simulink model "MSX60_10_by2"  (Simulink 7.9)
settings: Solver=ode14x  StartTime=0.0  StopTime=220  FixedStep=0.05  RelTol=1e-4
values from neighbouring files (symbols this model uses):
  G = yout(:,3)    [MSX60_10_by2_with_PandO.m]    (also in MSX60_10_by2_with_PandO_PS.m; MSX60_10_by2_with_PandO_US (1).m; MSX60_10_by2_with_PandO_US.m; MSX60_10by2Cell.m = 500)
  n = 1.3    [MSX60DS.m]    (also in MSX60_10_RL.m; MSX60_10_by2_with_PandO.m; MSX60_10_by2_with_PandO_PS.m; MSX60_10_by2_with_PandO_US (1).m)
  Ns = 1    [MSX60DS.m]    (also in MSX60_10_RL.m; MSX60_10_by2_with_PandO.m; MSX60_10_by2_with_PandO_PS.m; MSX60_10_by2_with_PandO_US (1).m)
  Rs = 0.58    [MSX60DS.m]    (also in MSX60_10_RL.m; MSX60_10_by2_with_PandO.m; MSX60_10_by2_with_PandO_PS.m; MSX60_10_by2_with_PandO_US (1).m)
  Voc = Voc(1)    [MSX60DS.m]    (also in MSX60_10_RL.m = 21.1; MSX60_10_by2_with_PandO.m = 21.1; MSX60_10_by2_with_PandO_PS.m = 21.1; MSX60_10_by2_with_PandO_US (1).m = 21.1)
libraries: fl_lib x23, elec_lib x20, nesl_utility x5, simulink x1
settings Model: Creator=pc1  LastModifiedBy=pc1
settings SolverCC: SolverJacobianMethodControl=SparsePerturbation
settings DataIOCC: SaveState=on

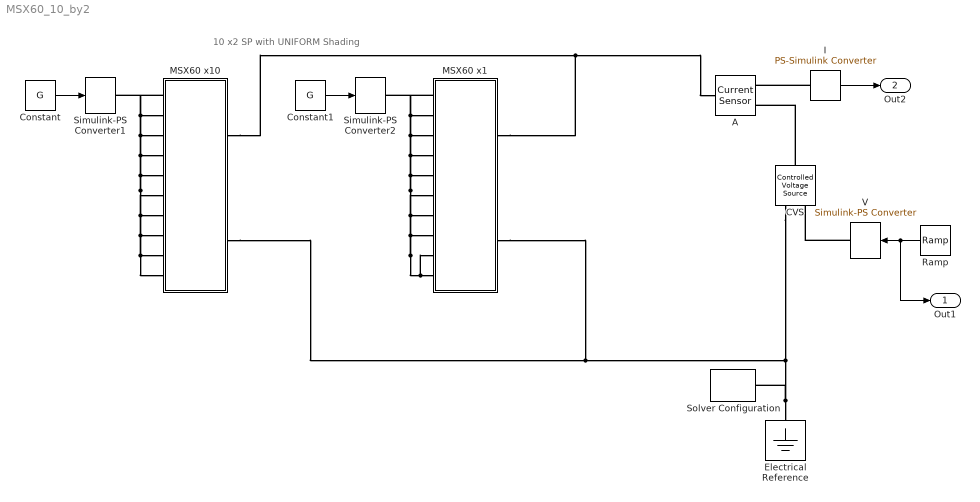
== system MSX60_10_by2 ==
  note: 10 x2 SP with UNIFORM Shading
  A : fl_lib/Electrical/Electrical Sensors/Current Sensor  i1_Log=off  v1_Log=off  LocalVarNames=|i1|v1  LocalVarDescs=|i1|v1  LocalVarLogging=[0 0]
  CVS : fl_lib/Electrical/Electrical Sources/Controlled Voltage Source  i_Log=off  v_Log=off  LocalVarNames=|i|v  LocalVarDescs=|i|v  LocalVarLogging=[0 0]
  Constant : Constant  Value=G
  Constant1 : Constant  Value=G
  Electrical Reference : fl_lib/Electrical/Electrical Elements/Electrical Reference  i_Log=off  LocalVarNames=|i  LocalVarDescs=|i  LocalVarLogging=0
  I : nesl_utility/PS-Simulink Converter  PhysicalDomain=network_engine_domain  LeftPortType=input  RightPortType=output  SubClassName=ps_output  Unit=1  AffineConversion=off
  MSX60 x1 : Subsystem
  MSX60 x10 : Subsystem
  Ramp : simulink/Sources/Ramp  slope=1  start=1  X0=0
  Simulink-PS Converter1 : nesl_utility/Simulink-PS Converter  PhysicalDomain=network_engine_domain  LeftPortType=input  RightPortType=output  SubClassName=ps_input  Unit=1  AffineConversion=off  InputFilterTimeConstant=.001  UdotUserProvided=[]  SimscapeFilterOrder=1  InputFiltering=off
  Simulink-PS Converter2 : nesl_utility/Simulink-PS Converter  PhysicalDomain=network_engine_domain  LeftPortType=input  RightPortType=output  SubClassName=ps_input  Unit=1  AffineConversion=off  InputFilterTimeConstant=.001  UdotUserProvided=[]  SimscapeFilterOrder=1  InputFiltering=off
  Solver Configuration : nesl_utility/Solver Configuration  PhysicalDomain=network_engine_domain  LeftPortType=input  RightPortType=generic  SubClassName=solver  UseCustomDae=off  DoDC=on  ResidualTolerance=1e-9  UseLocalSolver=off  LocalSolverChoice=NE_BACKWARD_EULER_ADVANCER  LocalSolverSampleTime=.001  DoFixedCost=off  MaxNonlinIter=3  MaxModeIter=2  LinearAlgebra=Sparse  Accelerate=off  Profile=off  UseLocalSampling=off  DelaysMemoryBudget=1024
  V : nesl_utility/Simulink-PS Converter  PhysicalDomain=network_engine_domain  LeftPortType=input  RightPortType=output  SubClassName=ps_input  Unit=1  AffineConversion=off  InputFilterTimeConstant=.001  UdotUserProvided=[]  SimscapeFilterOrder=1  InputFiltering=off
  Out1 : Outport
  Out2 : Outport  Port=2
  wires:
  I/1 -> Out2/1
  Ramp/1 -> V/1, Out1/1
  Constant/1 -> Simulink-PS Converter1/1
  Constant1/1 -> Simulink-PS Converter2/1
  connections:
  I/LConn1 -- A/RConn1
  MSX60 x10/RConn2 -- CVS/RConn2 -- Electrical Reference/LConn1 -- Solver Configuration/RConn1 -- MSX60 x1/RConn2
  CVS/LConn1 -- A/RConn2
  V/RConn1 -- CVS/RConn1
  MSX60 x10/LConn1 -- Simulink-PS Converter1/RConn1 -- MSX60 x10/LConn2 -- MSX60 x10/LConn3 -- MSX60 x10/LConn4 -- MSX60 x10/LConn5 -- MSX60 x10/LConn6 -- MSX60 x10/LConn7 -- MSX60 x10/LConn8 -- MSX60 x10/LConn9 -- MSX60 x10/LConn10
  MSX60 x1/LConn10 -- MSX60 x1/LConn1 -- Simulink-PS Converter2/RConn1 -- MSX60 x1/LConn2 -- MSX60 x1/LConn3 -- MSX60 x1/LConn4 -- MSX60 x1/LConn5 -- MSX60 x1/LConn6 -- MSX60 x1/LConn7 -- MSX60 x1/LConn8 -- MSX60 x1/LConn9
  MSX60 x10/RConn1 -- A/LConn1 -- MSX60 x1/RConn1

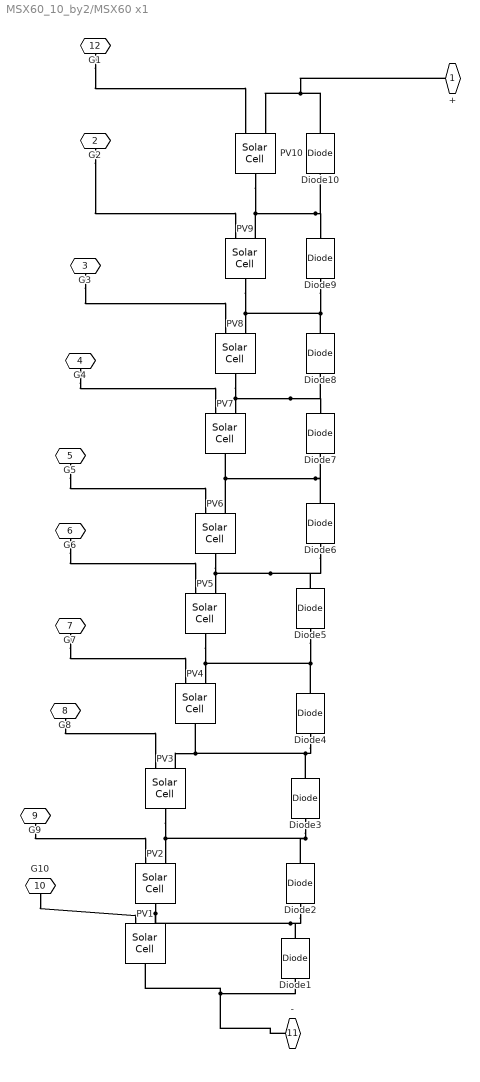
== system MSX60_10_by2/MSX60 x1 ==
  Diode{1..10} (10 alike) : fl_lib/Electrical/Electrical Elements/Diode  Vf=0.6 V  Ron=0.3 Ohm  Goff=1e-8 1/Ohm  i_Log=off  v_Log=off  LocalVarNames=|i|v  LocalVarDescs=|i|v  LocalVarLogging=[0 0]
  PV{1..10} (10 alike) : elec_lib/Sources/Solar Cell  prm=1  Isc=Isc A  Voc=Voc*Ns V  Is=1e-6 A  Is2=0 A  Iph=3.8 A  Ir0=Gstc W/m^2  ec=n*Voc*Ns  N2=0  Rs=Rs*Ns Ohm  Rp=Inf Ohm  TIPH1=0 1/K  EG=1.11 eV  TXIS1=3  TXIS2=3  TRS1=0  TRP1=0  Tmeas=25 C  TFIXED=25 C  LocalVarLogging=[]  thermal_mass=100 J/K  initial_temperature=25 C
  + : PMIOPort  Port=1  Side=Right
  G2 : PMIOPort  Port=2  Side=Left
  G3 : PMIOPort  Port=3  Side=Left
  G4 : PMIOPort  Port=4  Side=Left
  G5 : PMIOPort  Port=5  Side=Left
  G6 : PMIOPort  Port=6  Side=Left
  G7 : PMIOPort  Port=7  Side=Left
  G8 : PMIOPort  Port=8  Side=Left
  G9 : PMIOPort  Port=9  Side=Left
  G10 : PMIOPort  Port=10  Side=Left
  - : PMIOPort  Port=11  Side=Right
  G1 : PMIOPort  Port=12  Side=Left
  connections:
  Diode4/LConn1 -- PV3/LConn2 -- PV4/RConn1 -- Diode3/RConn1
  Diode5/LConn1 -- PV5/RConn1 -- PV4/LConn2 -- Diode4/RConn1
  Diode6/LConn1 -- PV6/RConn1 -- PV5/LConn2 -- Diode5/RConn1
  PV8/RConn1 -- PV7/LConn2 -- Diode7/RConn1 -- Diode8/LConn1
  Diode9/LConn1 -- PV8/LConn2 -- PV9/RConn1 -- Diode8/RConn1
  G10/RConn1 -- PV1/LConn1
  -/RConn1 -- PV1/RConn1 -- Diode1/LConn1
  G9/RConn1 -- PV2/LConn1
  Diode2/LConn1 -- PV2/RConn1 -- PV1/LConn2 -- Diode1/RConn1
  Diode3/LConn1 -- PV2/LConn2 -- PV3/RConn1 -- Diode2/RConn1
  G8/RConn1 -- PV3/LConn1
  PV6/LConn2 -- PV7/RConn1 -- Diode7/LConn1 -- Diode6/RConn1
  PV9/LConn2 -- PV10/RConn1 -- Diode9/RConn1 -- Diode10/LConn1
  Diode10/RConn1 -- PV10/LConn2 -- +/RConn1
  G7/RConn1 -- PV4/LConn1
  G6/RConn1 -- PV5/LConn1
  G5/RConn1 -- PV6/LConn1
  G4/RConn1 -- PV7/LConn1
  G3/RConn1 -- PV8/LConn1
  G2/RConn1 -- PV9/LConn1
  G1/RConn1 -- PV10/LConn1

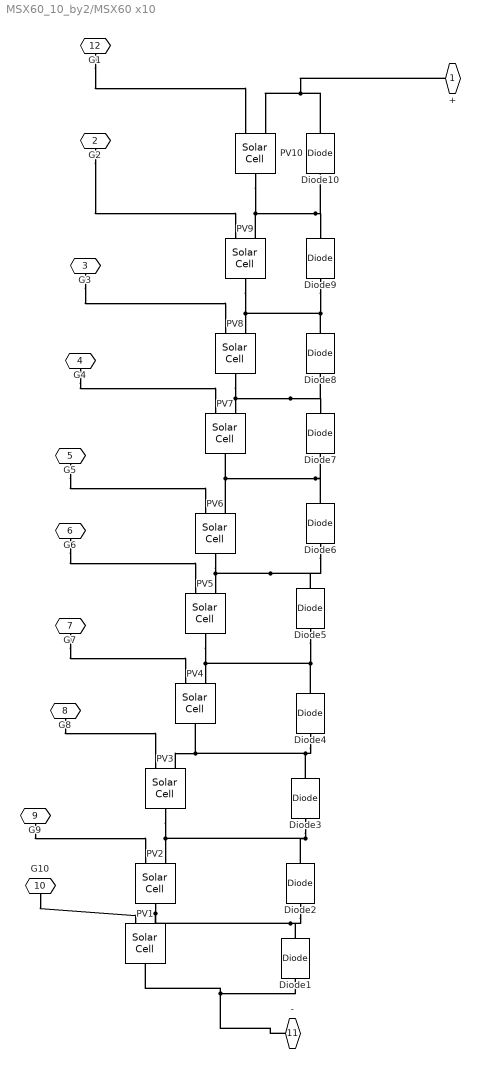
== system MSX60_10_by2/MSX60 x10 ==
  Diode{1..10} (10 alike) : fl_lib/Electrical/Electrical Elements/Diode  Vf=0.6 V  Ron=0.3 Ohm  Goff=1e-8 1/Ohm  i_Log=off  v_Log=off  LocalVarNames=|i|v  LocalVarDescs=|i|v  LocalVarLogging=[0 0]
  PV{1..10} (10 alike) : elec_lib/Sources/Solar Cell  prm=1  Isc=Isc A  Voc=Voc*Ns V  Is=1e-6 A  Is2=0 A  Iph=3.8 A  Ir0=Gstc W/m^2  ec=n*Voc*Ns  N2=0  Rs=Rs*Ns Ohm  Rp=Inf Ohm  TIPH1=0 1/K  EG=1.11 eV  TXIS1=3  TXIS2=3  TRS1=0  TRP1=0  Tmeas=25 C  TFIXED=25 C  LocalVarLogging=[]  thermal_mass=100 J/K  initial_temperature=25 C
  + : PMIOPort  Port=1  Side=Right
  G2 : PMIOPort  Port=2  Side=Left
  G3 : PMIOPort  Port=3  Side=Left
  G4 : PMIOPort  Port=4  Side=Left
  G5 : PMIOPort  Port=5  Side=Left
  G6 : PMIOPort  Port=6  Side=Left
  G7 : PMIOPort  Port=7  Side=Left
  G8 : PMIOPort  Port=8  Side=Left
  G9 : PMIOPort  Port=9  Side=Left
  G10 : PMIOPort  Port=10  Side=Left
  - : PMIOPort  Port=11  Side=Right
  G1 : PMIOPort  Port=12  Side=Left
  connections:
  Diode4/LConn1 -- PV3/LConn2 -- PV4/RConn1 -- Diode3/RConn1
  Diode5/LConn1 -- PV5/RConn1 -- PV4/LConn2 -- Diode4/RConn1
  Diode6/LConn1 -- PV6/RConn1 -- PV5/LConn2 -- Diode5/RConn1
  PV8/RConn1 -- PV7/LConn2 -- Diode7/RConn1 -- Diode8/LConn1
  Diode9/LConn1 -- PV8/LConn2 -- PV9/RConn1 -- Diode8/RConn1
  G10/RConn1 -- PV1/LConn1
  -/RConn1 -- PV1/RConn1 -- Diode1/LConn1
  G9/RConn1 -- PV2/LConn1
  Diode2/LConn1 -- PV2/RConn1 -- PV1/LConn2 -- Diode1/RConn1
  Diode3/LConn1 -- PV2/LConn2 -- PV3/RConn1 -- Diode2/RConn1
  G8/RConn1 -- PV3/LConn1
  PV6/LConn2 -- PV7/RConn1 -- Diode7/LConn1 -- Diode6/RConn1
  PV9/LConn2 -- PV10/RConn1 -- Diode9/RConn1 -- Diode10/LConn1
  Diode10/RConn1 -- PV10/LConn2 -- +/RConn1
  G7/RConn1 -- PV4/LConn1
  G6/RConn1 -- PV5/LConn1
  G5/RConn1 -- PV6/LConn1
  G4/RConn1 -- PV7/LConn1
  G3/RConn1 -- PV8/LConn1
  G2/RConn1 -- PV9/LConn1
  G1/RConn1 -- PV10/LConn1
